simulink model "d_039"  (Simulink 8.3)
settings: Solver=ode45  StartTime=0.0  StopTime=10.0  RelTol=1e-3
(part 2 of 2)

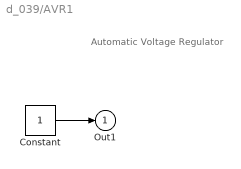
== system d_039/AVR1 ==
  note: Automatic Voltage Regulator
  Constant : Constant
  Out1 : Outport
  wires:
  Constant/1 -> Out1/1

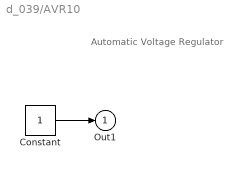
== system d_039/AVR10 ==
  note: Automatic Voltage Regulator
  Constant : Constant
  Out1 : Outport
  wires:
  Constant/1 -> Out1/1

== system d_039/AVR3 ==
  note: Automatic Voltage Regulator
  Constant : Constant
  Out1 : Outport
  wires:
  Constant/1 -> Out1/1

== system d_039/AVR4 ==
  note: Automatic Voltage Regulator
  Constant : Constant
  Out1 : Outport
  wires:
  Constant/1 -> Out1/1

== system d_039/AVR5 ==
  note: Automatic Voltage Regulator
  Constant : Constant
  Out1 : Outport
  wires:
  Constant/1 -> Out1/1

== system d_039/AVR6 ==
  note: Automatic Voltage Regulator
  Constant : Constant
  Out1 : Outport
  wires:
  Constant/1 -> Out1/1

== system d_039/AVR7 ==
  note: Automatic Voltage Regulator
  Constant : Constant
  Out1 : Outport
  wires:
  Constant/1 -> Out1/1

== system d_039/AVR8 ==
  note: Automatic Voltage Regulator
  Constant : Constant
  Out1 : Outport
  wires:
  Constant/1 -> Out1/1

== system d_039/AVR9 ==
  note: Automatic Voltage Regulator
  Constant : Constant
  Out1 : Outport
  wires:
  Constant/1 -> Out1/1

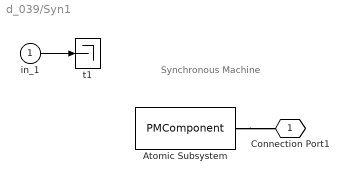
== system d_039/Syn1 ==
  note: Synchronous Machine
  in_1 : Inport
  Atomic Subsystem : PMComponent  PhysicalDomain=psatdomain  LeftPortType=p1  RightPortType=p1  RConnTagsString=__newr0
  t1 : Terminator
  Connection Port1 : PMIOPort  Tag=PMCPort  Port=1  Side=Right
  wires:
  in_1/1 -> t1/1
  connections:
  Atomic Subsystem/RConn1 -- Connection Port1/RConn1

== system d_039/Syn10 ==
  note: Synchronous Machine
  Atomic Subsystem : PMComponent  PhysicalDomain=psatdomain  LeftPortType=p1  RightPortType=p1  RConnTagsString=__newr0
  Connection Port1 : PMIOPort  Tag=PMCPort  Port=1  Side=Right
  connections:
  Atomic Subsystem/RConn1 -- Connection Port1/RConn1

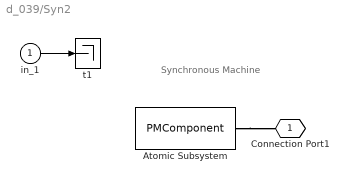
== system d_039/Syn2 ==
  note: Synchronous Machine
  in_1 : Inport
  Atomic Subsystem : PMComponent  PhysicalDomain=psatdomain  LeftPortType=p1  RightPortType=p1  RConnTagsString=__newr0
  t1 : Terminator
  Connection Port1 : PMIOPort  Tag=PMCPort  Port=1  Side=Right
  wires:
  in_1/1 -> t1/1
  connections:
  Atomic Subsystem/RConn1 -- Connection Port1/RConn1

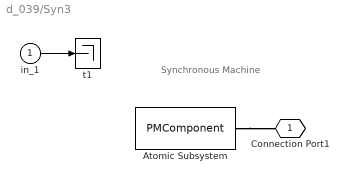
== system d_039/Syn3 ==
  note: Synchronous Machine
  in_1 : Inport
  Atomic Subsystem : PMComponent  PhysicalDomain=psatdomain  LeftPortType=p1  RightPortType=p1  RConnTagsString=__newr0
  t1 : Terminator
  Connection Port1 : PMIOPort  Tag=PMCPort  Port=1  Side=Right
  wires:
  in_1/1 -> t1/1
  connections:
  Atomic Subsystem/RConn1 -- Connection Port1/RConn1

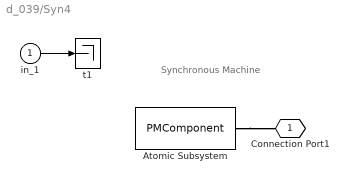
== system d_039/Syn4 ==
  note: Synchronous Machine
  in_1 : Inport
  Atomic Subsystem : PMComponent  PhysicalDomain=psatdomain  LeftPortType=p1  RightPortType=p1  RConnTagsString=__newr0
  t1 : Terminator
  Connection Port1 : PMIOPort  Tag=PMCPort  Port=1  Side=Right
  wires:
  in_1/1 -> t1/1
  connections:
  Atomic Subsystem/RConn1 -- Connection Port1/RConn1

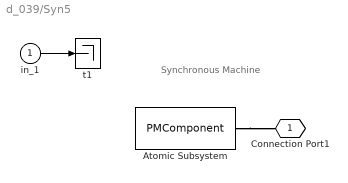
== system d_039/Syn5 ==
  note: Synchronous Machine
  in_1 : Inport
  Atomic Subsystem : PMComponent  PhysicalDomain=psatdomain  LeftPortType=p1  RightPortType=p1  RConnTagsString=__newr0
  t1 : Terminator
  Connection Port1 : PMIOPort  Tag=PMCPort  Port=1  Side=Right
  wires:
  in_1/1 -> t1/1
  connections:
  Atomic Subsystem/RConn1 -- Connection Port1/RConn1

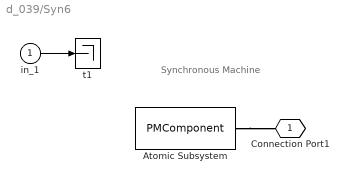
== system d_039/Syn6 ==
  note: Synchronous Machine
  in_1 : Inport
  Atomic Subsystem : PMComponent  PhysicalDomain=psatdomain  LeftPortType=p1  RightPortType=p1  RConnTagsString=__newr0
  t1 : Terminator
  Connection Port1 : PMIOPort  Tag=PMCPort  Port=1  Side=Right
  wires:
  in_1/1 -> t1/1
  connections:
  Atomic Subsystem/RConn1 -- Connection Port1/RConn1

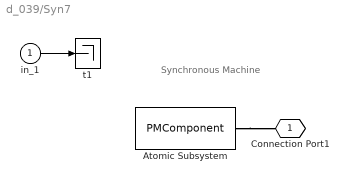
== system d_039/Syn7 ==
  note: Synchronous Machine
  in_1 : Inport
  Atomic Subsystem : PMComponent  PhysicalDomain=psatdomain  LeftPortType=p1  RightPortType=p1  RConnTagsString=__newr0
  t1 : Terminator
  Connection Port1 : PMIOPort  Tag=PMCPort  Port=1  Side=Right
  wires:
  in_1/1 -> t1/1
  connections:
  Atomic Subsystem/RConn1 -- Connection Port1/RConn1

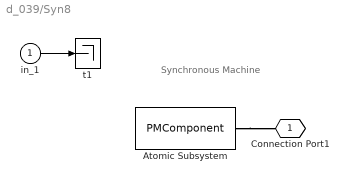
== system d_039/Syn8 ==
  note: Synchronous Machine
  in_1 : Inport
  Atomic Subsystem : PMComponent  PhysicalDomain=psatdomain  LeftPortType=p1  RightPortType=p1  RConnTagsString=__newr0
  t1 : Terminator
  Connection Port1 : PMIOPort  Tag=PMCPort  Port=1  Side=Right
  wires:
  in_1/1 -> t1/1
  connections:
  Atomic Subsystem/RConn1 -- Connection Port1/RConn1

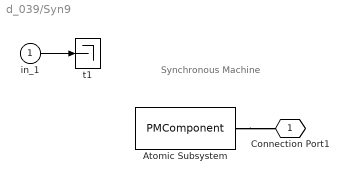
== system d_039/Syn9 ==
  note: Synchronous Machine
  in_1 : Inport
  Atomic Subsystem : PMComponent  PhysicalDomain=psatdomain  LeftPortType=p1  RightPortType=p1  RConnTagsString=__newr0
  t1 : Terminator
  Connection Port1 : PMIOPort  Tag=PMCPort  Port=1  Side=Right
  wires:
  in_1/1 -> t1/1
  connections:
  Atomic Subsystem/RConn1 -- Connection Port1/RConn1
